simulink model "sf_array"  (Simulink 6.0)
settings: Solver=ode45  StartTime=0  StopTime=1  MaxStep=1  RelTol=1e-3
settings Model: CovMetricSettings=dcmtr  Creator=The MathWorks Inc.  LastModifiedBy=batserve  ExtModeAutoUpdateStatusClock=off
settings DataIOCC: SignalLoggingName=sigsOut
settings OptimizationCC: BooleanDataType=off
settings DebuggingCC: CheckExecutionContextPreStartOutputMsg=on  CheckExecutionContextRuntimeOutputMsg=on  SolverPrmCheckMsg=none
settings HardwareCC: TargetUnknown=on

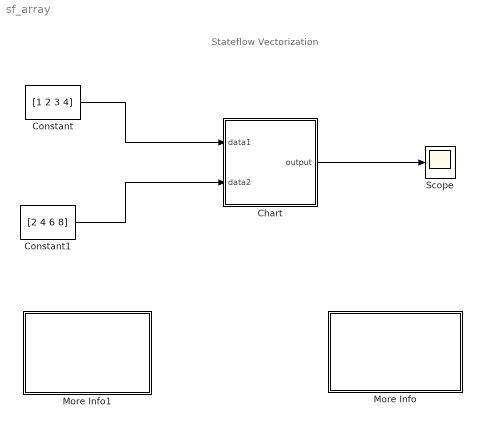
== system sf_array ==
  note: Stateflow Vectorization
  Chart : Stateflow chart  PropExecContextAcrossSSBoundary=on
  Constant : Constant  Value=[1 2 3 4]
  Constant1 : Constant  Value=[2 4 6 8]
  More Info : Subsystem  PropExecContextAcrossSSBoundary=on
      mask Display: disp('Double click\nhere for\ninformation on\nthis demonstration')
  More Info1 : Subsystem  PropExecContextAcrossSSBoundary=on
      settings: OpenFcn=simcad(bdroot);
      mask Display: disp('Double click\nhere for\nSimulink\Stateflow\n Help')
  Scope : Scope
      settings: YMin=0  YMax=55
  wires:
  Constant/1 -> Chart/1(data1)
  Constant1/1 -> Chart/2(data2)
  Chart/1(output) -> Scope/1

== system sf_array/More Info ==
  note: Vectorization
  note: Stateflow has the ability to vectorize the data inputs and perform 1-D array manipulations. In this example,
      | the following MATLAB code is implemented:
      |
      | data1=[1 2 3 4];
      | data2=[2 4 6 8];
      | output=data1.*data2+1;
      |
      | Notice the array operator '.' placed before the multiplication sign. Stateflow also implements this vectorization
      | which eliminates the need for DO or FOR loops. The reult is a faster, more efficient code that is also easier to
      | implement.

== system sf_array/More Info1 ==

== stateflow chart Chart ==
  note: Equivalent MATLAB code:
      |
      | data1=[1 2 3 4];
      | data2=[2 4 6 8];
      | output=data1.*data2+1;
  (default) -> (junction 4) : {output=data1*data2 + 1;}
  data: output output double size=4; data1 input double size=4; data2 input double size=4
